simulink model "maddparam"  (Simulink 7.6)
settings: Solver=FixedStepDiscrete  StartTime=0.0  StopTime=10.0  RelTol=1e-3
settings Model: NewParam1=value1  NewParam2=value2  Creator=mtocci  LastModifiedBy=mtocci
settings OptimizationCC: InlineParams=on

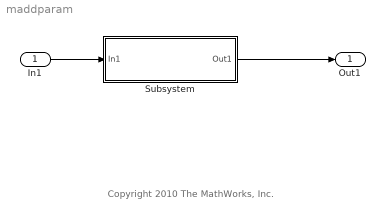
== system maddparam ==
  note: Copyright 2010 The MathWorks, Inc.
  In1 : Inport
  Subsystem : Subsystem  TreatAsAtomicUnit=on
  Out1 : Outport
  wires:
  In1/1 -> Subsystem/1(In1)
  Subsystem/1(Out1) -> Out1/1

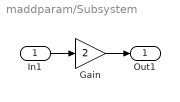
== system maddparam/Subsystem ==
  In1 : Inport
  Gain : Gain  Gain=2  ParameterDataType=fixdt(1, 16)  ParameterScaling=2^0  OutDataType=fixdt(1, 16)  OutScaling=2^0
  Out1 : Outport
  wires:
  In1/1 -> Gain/1
  Gain/1 -> Out1/1
